simulink model "test_save_vector"  (R2024a)
settings: Solver=VariableStepAuto  StartTime=0.0  StopTime=10.0  RelTol=1e-3
settings Model: SimulationMode=accelerator  Creator=thatf  LastModifiedBy=thatf

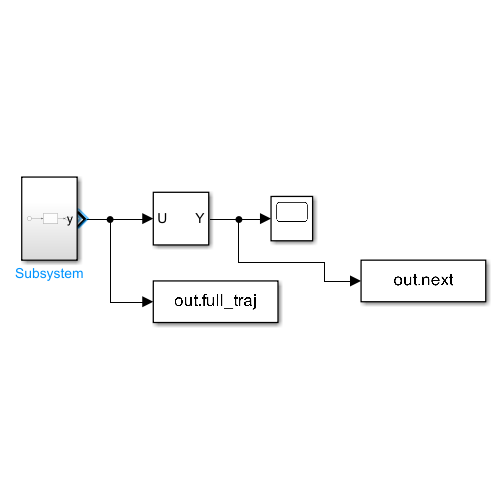
[thumbnail: Simulink's stored preview of the top-level diagram]
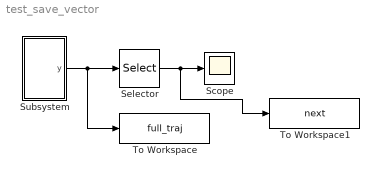
== system test_save_vector ==
  Scope : Scope
  Selector : Selector  NumberOfDimensions=2  InputPortWidth=3  IndexOptions=Index vector (dialog),Select all  Indices=[1],1  OutputSizes=1,1
  Subsystem : Subsystem
  To Workspace : ToWorkspace  VariableName=full_traj  SampleTime=-1
  To Workspace1 : ToWorkspace  VariableName=next  SampleTime=-1
  wires:
  Subsystem/1(y) -> To Workspace/1, Selector/1
  Selector/1 -> To Workspace1/1, Scope/1

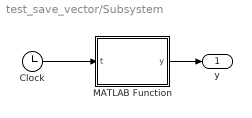
== system test_save_vector/Subsystem ==
  Clock : Clock
  MATLAB Function : MATLAB Function  TreatAsAtomicUnit=on
  y : Outport
  wires:
  Clock/1 -> MATLAB Function/1(t)
  MATLAB Function/1(y) -> y/1

== matlab function test_save_vector/Subsystem/MATLAB Function ==
  data: t input; y output
function y = fcn(t)

y = [1 -1; 2 -2; 3 -3; 4 -4; 5 -5] + t;
